simulink model "glitch_filter"  (R2021a)
settings: Solver=FixedStepDiscrete  StartTime=0.0  StopTime=10.0  RelTol=1e-3
PreLoadFcn:
  | addpath('C:\Repo_TESIS_verilog\Tesis-LGBS\Matlab\hdlimport\glitch_filter');
CloseFcn:
  | addpath('C:\Repo_TESIS_verilog\Tesis-LGBS\Matlab\hdlimport\glitch_filter');
  | rmpath('C:\Repo_TESIS_verilog\Tesis-LGBS\Matlab\hdlimport\glitch_filter');
settings Model: DataTypeOverride=Off  Creator=Damian  LastModifiedBy=Damian
settings OptimizationCC: BlockReduction=off  ConditionallyExecuteInputs=off  DefaultParameterBehavior=Inlined
settings DebuggingCC: AlgebraicLoopMsg=error  InheritedTsInSrcMsg=none  SingleTaskRateTransMsg=error
settings HardwareCC: ProdBitPerPointer=32  ProdBitPerSizeT=32  ProdBitPerPtrDiffT=32  ProdLargestAtomicFloat=None  ProdIntDivRoundTo=Undefined  ProdEndianess=Unspecified  ProdWordSize=32  ProdHWDeviceType=ASIC/FPGA->ASIC/FPGA  TargetBitPerPointer=64  TargetBitPerSizeT=64  TargetBitPerPtrDiffT=64  TargetLongLongMode=on  TargetIntDivRoundTo=Zero  TargetEndianess=LittleEndian  TargetWordSize=64  TargetHWDeviceType=Custom Processor->MATLAB Host Computer  ProdEqTarget=off

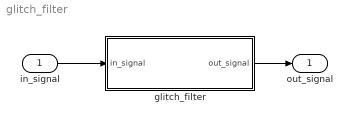
== system glitch_filter ==
  in_signal : Inport  OutDataTypeStr=fixdt(0, 6, 0)  SampleTime=-1
  glitch_filter : Subsystem
  out_signal : Outport  OutDataTypeStr=fixdt(0, 6, 0)  SampleTime=-1
  wires:
  glitch_filter/1(out_signal) -> out_signal/1
  in_signal/1 -> glitch_filter/1(in_signal)

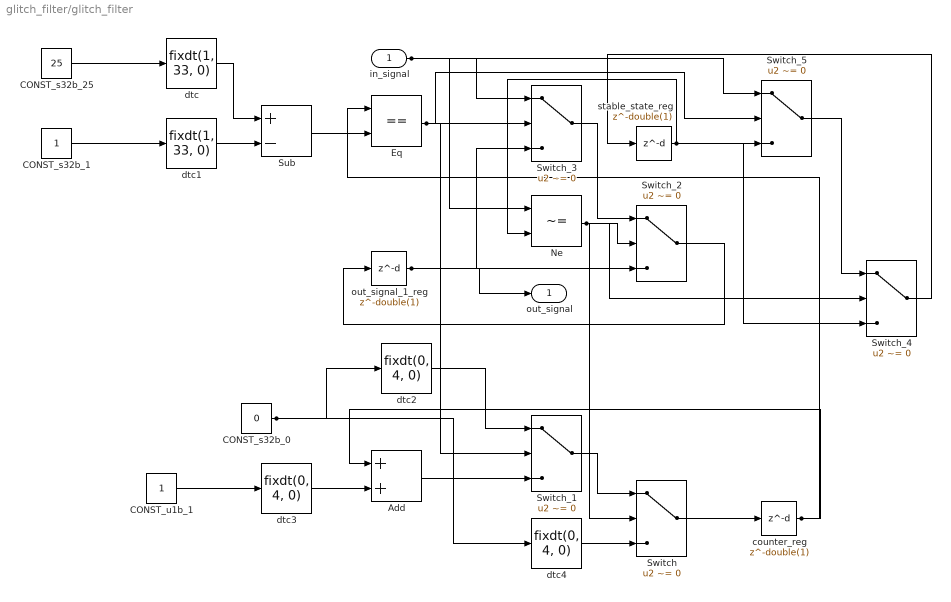
== system glitch_filter/glitch_filter ==
  in_signal : Inport  OutDataTypeStr=fixdt(0, 6, 0)  SampleTime=-1
  Add : Sum  AccumDataTypeStr=fixdt(0, 4, 0)  OutDataTypeStr=fixdt(0, 4, 0)  SampleTime=-1
  CONST_s32b_0 : Constant  Value=0  OutDataTypeStr=int32  SampleTime=-1
  CONST_s32b_1 : Constant  OutDataTypeStr=int32  SampleTime=-1
  CONST_s32b_25 : Constant  Value=25  OutDataTypeStr=int32  SampleTime=-1
  CONST_u1b_1 : Constant  OutDataTypeStr=fixdt(0, 1, 0)  SampleTime=-1
  Eq : RelationalOperator  Operator===  OutDataTypeStr=fixdt(0,1,0)  SampleTime=-1  RndMeth=Nearest
  Ne : RelationalOperator  Operator=~=  OutDataTypeStr=fixdt(0,1,0)  SampleTime=-1  RndMeth=Nearest
  Sub : Sum  Inputs=+-  AccumDataTypeStr=fixdt(1, 33, 0)  OutDataTypeStr=fixdt(1, 33, 0)  SampleTime=-1
  Switch : Switch  Criteria=u2 ~= 0  Threshold=double(0)  OutDataTypeStr=fixdt(0, 4, 0)  SampleTime=-1
  Switch_1 : Switch  Criteria=u2 ~= 0  Threshold=double(0)  OutDataTypeStr=fixdt(0, 4, 0)  SampleTime=-1
  Switch_{2..5} (4 alike) : Switch  Criteria=u2 ~= 0  Threshold=double(0)  OutDataTypeStr=fixdt(0, 6, 0)  SampleTime=-1
  counter_reg : Delay  DelayLength=double(1)  InitialCondition=0  SampleTime=-1
  dtc : DataTypeConversion  OutDataTypeStr=fixdt(1, 33, 0)  SampleTime=-1
  dtc1 : DataTypeConversion  OutDataTypeStr=fixdt(1, 33, 0)  SampleTime=-1
  dtc2 : DataTypeConversion  OutDataTypeStr=fixdt(0, 4, 0)  SampleTime=-1
  dtc3 : DataTypeConversion  OutDataTypeStr=fixdt(0, 4, 0)  SampleTime=-1
  dtc4 : DataTypeConversion  OutDataTypeStr=fixdt(0, 4, 0)  SampleTime=-1
  out_signal_1_reg : Delay  DelayLength=double(1)  InitialCondition=0  SampleTime=-1
  stable_state_reg : Delay  DelayLength=double(1)  InitialCondition=0  SampleTime=-1
  out_signal : Outport  OutDataTypeStr=fixdt(0, 6, 0)  SampleTime=-1
  wires:
  Sub/1 -> Eq/2
  dtc2/1 -> Switch_1/1
  Switch_3/1 -> Switch_2/1
  Switch_5/1 -> Switch_4/1
  dtc4/1 -> Switch/3
  Add/1 -> Switch_1/3
  dtc3/1 -> Add/2
  CONST_u1b_1/1 -> dtc3/1
  dtc1/1 -> Sub/2
  Switch_1/1 -> Switch/1
  Switch/1 -> counter_reg/1
  CONST_s32b_1/1 -> dtc1/1
  Switch_4/1 -> stable_state_reg/1
  Switch_2/1 -> out_signal_1_reg/1
  dtc/1 -> Sub/1
  CONST_s32b_25/1 -> dtc/1
  Eq/1 -> Switch_5/2, Switch_3/2, Switch_1/2
  Ne/1 -> Switch_4/2, Switch_2/2, Switch/2
  counter_reg/1 -> Add/1, Eq/1
  CONST_s32b_0/1 -> dtc4/1, dtc2/1
  stable_state_reg/1 -> Switch_5/3, Switch_4/3, Ne/2
  out_signal_1_reg/1 -> Switch_3/3, Switch_2/3, out_signal/1
  in_signal/1 -> Switch_5/1, Switch_3/1, Ne/1
